simulink model "ex1"  (R2016a)
settings: Solver=ode3  StartTime=0.0  StopTime=inf  FixedStep=0.05  RelTol=1e-3
libraries: dsparch4 x4, simulink x3, vrlib x1, sldrtlib x1
settings Model: ExtModeTrigDuration=100000  Creator=kdle  LastModifiedBy=Khoa
settings DataIOCC: LimitDataPoints=on  SaveFormat=Array
settings DebuggingCC: UnderspecifiedInitializationDetection=Classic  MergeDetectMultiDrivingBlocksExec=none  SolverPrmCheckMsg=warning  StateNameClashWarn=warning
settings HardwareCC: ProdBitPerPointer=32  ProdLargestAtomicFloat=None  ProdIntDivRoundTo=Undefined  ProdEndianess=Unspecified  ProdWordSize=32  ProdHWDeviceType=32-bit Generic
settings ModelReferenceCC: PropagateSignalLabelsOutOfModel=off
settings ConfigComp: CovModelRefEnable=Off

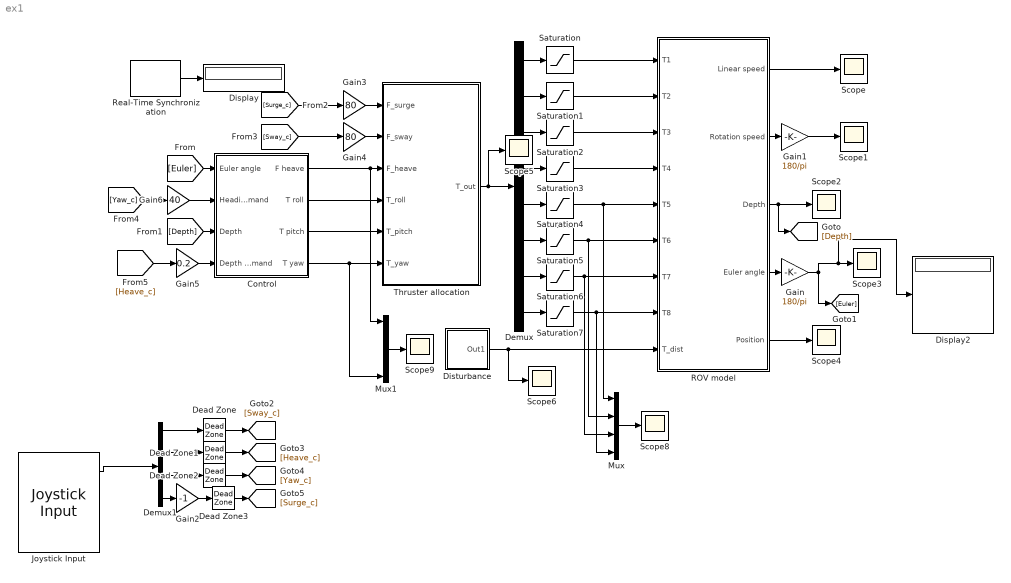
== system ex1 ==
  Control : Subsystem
  Dead Zone{,1..3} (4 alike) : DeadZone  LowerValue=-0.1  UpperValue=0.1  SaturateOnIntegerOverflow=on
  Demux : Demux  Outputs=8
  Demux1 : Demux
  Display : Display
  Display2 : Display
  Disturbance : Subsystem
  Gain : Gain  Gain=180/pi
  Gain1 : Gain  Gain=180/pi
  Gain2 : Gain  Gain=-1
  Gain3 : Gain  Gain=80
  Gain4 : Gain  Gain=80
  Gain5 : Gain  Gain=0.2
  Gain6 : Gain  Gain=40
  Joystick Input : vrlib/Joystick Input  joyid=1  adjustports=on  forcefeed=off
  Mux : Mux
  Mux1 : Mux
  ROV model : Subsystem
  Real-Time Synchronization : sldrtlib/Real-Time Synchronization  SampleTime=0.05  MaxMissedTicks=10000  ShowMissedTicks=on  YieldWhenWaiting=off
  Saturation{,1..3} (4 alike) : Saturate  UpperLimit=50  LowerLimit=-50
  Saturation{4..7} (4 alike) : Saturate  UpperLimit=20  LowerLimit=-20
  Scope{,1..6,8..9} (9 alike) : Scope
  Thruster allocation : MATLAB Function  TreatAsAtomicUnit=on
  wires:
  ROV model/1(Linear speed) -> Scope/1
  ROV model/2(Rotation speed) -> Gain1/1
  ROV model/3(Depth) -> [Depth], Scope2/1
  Disturbance/1(Out1) -> Scope6/1, ROV model/9(T_dist)
  ROV model/4(Euler angle) -> Gain/1
  Thruster allocation/1(T_out) -> Scope5/1, Demux/1
  Demux/7 -> Saturation6/1
  Demux/6 -> Saturation5/1
  Demux/8 -> Saturation7/1
  Demux/5 -> Saturation4/1
  Demux/4 -> Saturation3/1
  Demux/3 -> Saturation2/1
  Demux/2 -> Saturation1/1
  Demux/1 -> Saturation/1
  ROV model/5(Position) -> Scope4/1
  [Euler] -> Control/1(Euler angle)
  [Depth] -> Control/3(Depth)
  [Yaw_c] -> Gain6/1
  [Heave_c] -> Gain5/1
  Gain/1 -> Display2/1, Scope3/1, [Euler]
  Gain1/1 -> Scope1/1
  Saturation/1 -> ROV model/1(T1)
  Saturation1/1 -> ROV model/2(T2)
  Saturation2/1 -> ROV model/3(T3)
  Saturation3/1 -> ROV model/4(T4)
  Saturation4/1 -> Mux/1, ROV model/5(T5)
  Saturation5/1 -> Mux/2, ROV model/6(T6)
  Saturation6/1 -> Mux/3, ROV model/7(T7)
  Saturation7/1 -> Mux/4, ROV model/8(T8)
  Control/1(F heave) -> Mux1/1, Thruster allocation/3(F_heave)
  Control/4(T yaw) -> Mux1/4, Thruster allocation/6(T_yaw)
  Mux/1 -> Scope8/1
  Mux1/1 -> Scope9/1
  Real-Time Synchronization/1 -> Display/1
  Joystick Input/1 -> Demux1/1
  Demux1/1 -> Dead Zone/1
  Demux1/2 -> Dead Zone1/1
  Demux1/3 -> Dead Zone2/1
  Demux1/4 -> Gain2/1
  Gain3/1 -> Thruster allocation/1(F_surge)
  [Surge_c] -> Gain3/1
  [Sway_c] -> Gain4/1
  Gain4/1 -> Thruster allocation/2(F_sway)
  Dead Zone/1 -> [Sway_c]
  Dead Zone1/1 -> [Heave_c]
  Dead Zone2/1 -> [Yaw_c]
  Gain2/1 -> Dead Zone3/1
  Dead Zone3/1 -> [Surge_c]
  Gain5/1 -> Control/4(Depth Command)
  Gain6/1 -> Control/2(Heading Command)
  Control/2(T roll) -> Thruster allocation/4(T_roll)
  Control/3(T pitch) -> Thruster allocation/5(T_pitch)

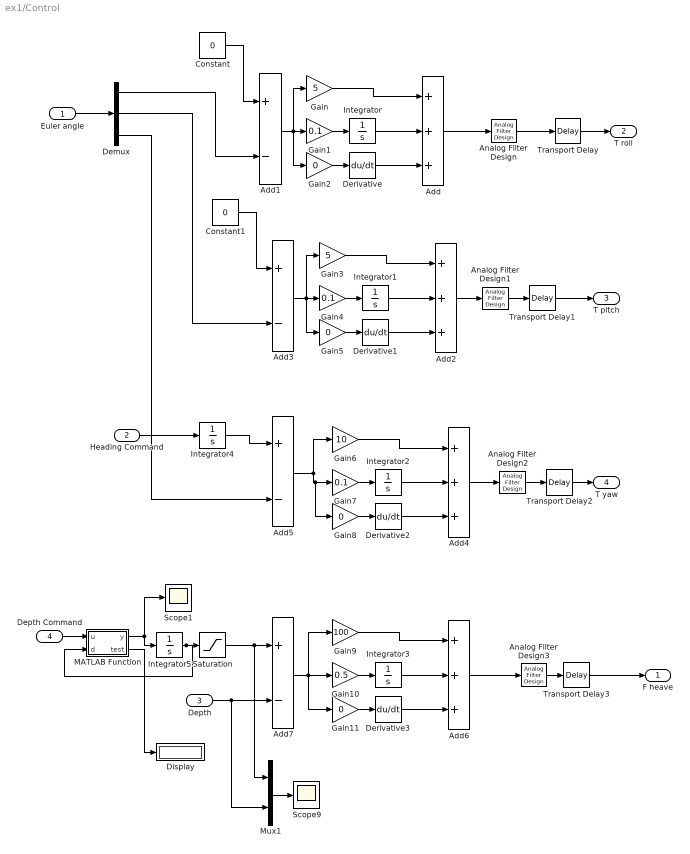
== system ex1/Control ==
  Euler angle : Inport
  Heading Command : Inport  Port=2
  Depth : Inport  Port=3
  Depth Command : Inport  Port=4
  Add{,2,4,6} (4 alike) : Sum  Inputs=+++
  Add{1,3,5,7} (4 alike) : Sum  Inputs=+-
  Analog Filter Design{,1..3} (4 alike) : dsparch4/Analog Filter Design  method=Butterworth  filttype=Lowpass  N=1  Wlo=20  Whi=80  Rp=2  Rs=40
  Constant : Constant  Value=0
  Constant1 : Constant  Value=0
  Demux : Demux  Outputs=3
  Derivative{,1..3} (4 alike) : Derivative
  Display : Display
  Gain : Gain  Gain=5
  Gain1 : Gain  Gain=0.1
  Gain10 : Gain  Gain=0.5
  Gain{2,5,8,11} (4 alike) : Gain  Gain=0
  Gain3 : Gain  Gain=5
  Gain4 : Gain  Gain=0.1
  Gain6 : Gain  Gain=10
  Gain7 : Gain  Gain=0.1
  Gain9 : Gain  Gain=100
  Integrator{,1..4} (5 alike) : Integrator
  Integrator5 : Integrator  InitialCondition=0.01
  MATLAB Function : MATLAB Function  TreatAsAtomicUnit=on
  Mux1 : Mux  Inputs=2
  Saturation : Saturate  UpperLimit=5  LowerLimit=0
  Scope1 : Scope
  Scope9 : Scope
  Transport Delay{,1..3} (4 alike) : TransportDelay  DelayTime=0
  F heave : Outport
  T roll : Outport  Port=2
  T pitch : Outport  Port=3
  T yaw : Outport  Port=4
  wires:
  Euler angle/1 -> Demux/1
  Gain1/1 -> Integrator/1
  Gain2/1 -> Derivative/1
  Gain/1 -> Add/1
  Integrator/1 -> Add/2
  Derivative/1 -> Add/3
  Add1/1 -> Gain2/1, Gain/1, Gain1/1
  Demux/1 -> Add1/2
  Constant/1 -> Add1/1
  Add/1 -> Analog Filter Design/1
  Gain4/1 -> Integrator1/1
  Gain5/1 -> Derivative1/1
  Gain3/1 -> Add2/1
  Integrator1/1 -> Add2/2
  Derivative1/1 -> Add2/3
  Add3/1 -> Gain4/1, Gain3/1, Gain5/1
  Demux/2 -> Add3/2
  Constant1/1 -> Add3/1
  Add2/1 -> Analog Filter Design1/1
  Gain7/1 -> Integrator2/1
  Gain8/1 -> Derivative2/1
  Gain6/1 -> Add4/1
  Integrator2/1 -> Add4/2
  Derivative2/1 -> Add4/3
  Gain10/1 -> Integrator3/1
  Gain11/1 -> Derivative3/1
  Gain9/1 -> Add6/1
  Integrator3/1 -> Add6/2
  Derivative3/1 -> Add6/3
  Add6/1 -> Analog Filter Design3/1
  Analog Filter Design/1 -> Transport Delay/1
  Analog Filter Design1/1 -> Transport Delay1/1
  Analog Filter Design2/1 -> Transport Delay2/1
  Analog Filter Design3/1 -> Transport Delay3/1
  Add4/1 -> Analog Filter Design2/1
  Transport Delay/1 -> T roll/1
  Transport Delay1/1 -> T pitch/1
  Transport Delay2/1 -> T yaw/1
  Transport Delay3/1 -> F heave/1
  Add5/1 -> Gain6/1, Gain8/1, Gain7/1
  Add7/1 -> Gain11/1, Gain9/1, Gain10/1
  Demux/3 -> Add5/2
  Heading Command/1 -> Integrator4/1
  Integrator4/1 -> Add5/1
  Depth/1 -> Mux1/2, Add7/2
  MATLAB Function/1(y) -> Integrator5/1, Scope1/1
  Depth Command/1 -> MATLAB Function/1(u)
  Integrator5/1 -> MATLAB Function/2(d), Saturation/1
  Mux1/1 -> Scope9/1
  Saturation/1 -> Mux1/1, Add7/1
  MATLAB Function/2(test) -> Display/1

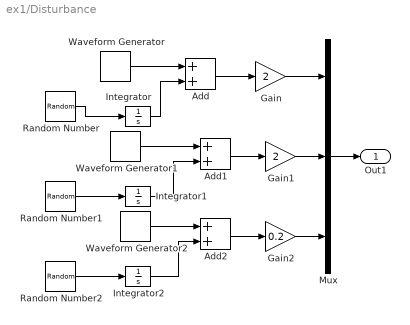
== system ex1/Disturbance ==
  Add : Sum
  Add1 : Sum
  Add2 : Sum
  Gain : Gain  Gain=2
  Gain1 : Gain  Gain=2
  Gain2 : Gain  Gain=0.2
  Integrator : Integrator
  Integrator1 : Integrator
  Integrator2 : Integrator
  Mux : Mux  Inputs=3
  Random Number : RandomNumber  Variance=4
  Random Number1 : RandomNumber  Variance=3.5  Seed=19
  Random Number2 : RandomNumber  Variance=2.7  Seed=12
  Waveform Generator : simulink/Sources/Waveform Generator  OutMin=[]  OutMax=[]  OutDataTypeStr=double  SelectedSignal=1  Signals=sin(9,0.8,1)+sin(3,1,90)+sin(0.5,2.3,150)#  BlockNames=MultiportSwitch_466ab8b035bb466#MultiportSwitch_63944deda71346d  SampleTime=-1
  Waveform Generator1 : simulink/Sources/Waveform Generator  OutMin=[]  OutMax=[]  OutDataTypeStr=double  SelectedSignal=1  Signals=sin(10,0.9,-80)+sin(3.5,1.2,90)+sin(0.5,2,180)##  BlockNames=MultiportSwitch_830e07a5a85d43f#MultiportSwitch_1fa4dfc1fb8347c#MultiportSwitch_a18988079fe14e6  SampleTime=-1
  Waveform Generator2 : simulink/Sources/Waveform Generator  OutMin=[]  OutMax=[]  OutDataTypeStr=double  SelectedSignal=1  Signals=sin(7,1.1,-80)+sin(3.4,1.6,85)+sin(0.5,2,180)##  BlockNames=MultiportSwitch_b1ec6a342e4a44b#MultiportSwitch_f195588b21b946e#MultiportSwitch_f4c491ab188140c  SampleTime=-1
  Out1 : Outport
  wires:
  Mux/1 -> Out1/1
  Waveform Generator/1 -> Add/1
  Add/1 -> Gain/1
  Add1/1 -> Gain1/1
  Waveform Generator1/1 -> Add1/1
  Add2/1 -> Gain2/1
  Waveform Generator2/1 -> Add2/1
  Random Number/1 -> Integrator/1
  Random Number1/1 -> Integrator1/1
  Random Number2/1 -> Integrator2/1
  Integrator/1 -> Add/2
  Integrator1/1 -> Add1/2
  Integrator2/1 -> Add2/2
  Gain/1 -> Mux/1
  Gain1/1 -> Mux/2
  Gain2/1 -> Mux/3

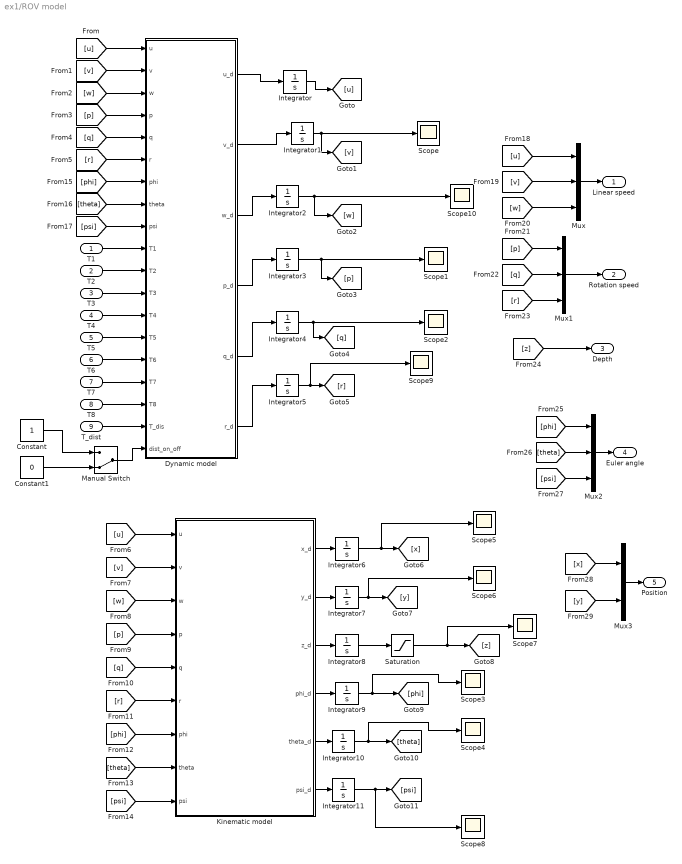
== system ex1/ROV model ==
  T1 : Inport
  T2 : Inport  Port=2
  T3 : Inport  Port=3
  T4 : Inport  Port=4
  T5 : Inport  Port=5
  T6 : Inport  Port=6
  T7 : Inport  Port=7
  T8 : Inport  Port=8
  T_dist : Inport  Port=9
  Constant : Constant
  Constant1 : Constant  Value=0
  Dynamic model : MATLAB Function  TreatAsAtomicUnit=on
  Integrator{,1..11} (12 alike) : Integrator
  Kinematic model : MATLAB Function  TreatAsAtomicUnit=on
  Manual Switch : ManualSwitch  CurrentSetting=0
  Mux : Mux  Inputs=3
  Mux1 : Mux  Inputs=3
  Mux2 : Mux  Inputs=3
  Mux3 : Mux  Inputs=2
  Saturation : Saturate  UpperLimit=5  LowerLimit=0
  Scope{,1..10} (11 alike) : Scope
  Linear speed : Outport
  Rotation speed : Outport  Port=2
  Depth : Outport  Port=3
  Euler angle : Outport  Port=4
  Position : Outport  Port=5
  wires:
  T1/1 -> Dynamic model/10(T1)
  T2/1 -> Dynamic model/11(T2)
  T3/1 -> Dynamic model/12(T3)
  Dynamic model/1(u_d) -> Integrator/1
  Dynamic model/2(v_d) -> Integrator1/1
  Dynamic model/3(w_d) -> Integrator2/1
  Dynamic model/4(p_d) -> Integrator3/1
  Dynamic model/5(q_d) -> Integrator4/1
  Dynamic model/6(r_d) -> Integrator5/1
  Integrator/1 -> [u]
  Integrator1/1 -> [v], Scope/1
  Integrator2/1 -> [w], Scope10/1
  Integrator3/1 -> [p], Scope1/1
  Integrator4/1 -> [q], Scope2/1
  Integrator5/1 -> Scope9/1, [r]
  [u] -> Dynamic model/1(u)
  [v] -> Dynamic model/2(v)
  [w] -> Dynamic model/3(w)
  [p] -> Dynamic model/4(p)
  [r] -> Dynamic model/6(r)
  [q] -> Dynamic model/5(q)
  [u] -> Kinematic model/1(u)
  [r] -> Kinematic model/6(r)
  [q] -> Kinematic model/5(q)
  [p] -> Kinematic model/4(p)
  [w] -> Kinematic model/3(w)
  [v] -> Kinematic model/2(v)
  Kinematic model/1(x_d) -> Integrator6/1
  Kinematic model/2(y_d) -> Integrator7/1
  Kinematic model/3(z_d) -> Integrator8/1
  Kinematic model/4(phi_d) -> Integrator9/1
  Kinematic model/5(theta_d) -> Integrator10/1
  Kinematic model/6(psi_d) -> Integrator11/1
  Integrator6/1 -> Scope5/1, [x]
  Integrator7/1 -> Scope6/1, [y]
  Integrator8/1 -> Saturation/1
  Integrator9/1 -> Scope3/1, [phi]
  Integrator10/1 -> Scope4/1, [theta]
  Integrator11/1 -> Scope8/1, [psi]
  [phi] -> Kinematic model/7(phi)
  [theta] -> Kinematic model/8(theta)
  [psi] -> Kinematic model/9(psi)
  [phi] -> Dynamic model/7(phi)
  [theta] -> Dynamic model/8(theta)
  T4/1 -> Dynamic model/13(T4)
  T5/1 -> Dynamic model/14(T5)
  T6/1 -> Dynamic model/15(T6)
  T7/1 -> Dynamic model/16(T7)
  T8/1 -> Dynamic model/17(T8)
  [psi] -> Dynamic model/9(psi)
  T_dist/1 -> Dynamic model/18(T_dis)
  [u] -> Mux/1
  [v] -> Mux/2
  [w] -> Mux/3
  Mux/1 -> Linear speed/1
  [p] -> Mux1/1
  [q] -> Mux1/2
  [r] -> Mux1/3
  Mux1/1 -> Rotation speed/1
  [z] -> Depth/1
  Mux2/1 -> Euler angle/1
  [phi] -> Mux2/1
  [theta] -> Mux2/2
  [psi] -> Mux2/3
  Mux3/1 -> Position/1
  [x] -> Mux3/1
  [y] -> Mux3/2
  Saturation/1 -> Scope7/1, [z]
  Manual Switch/1 -> Dynamic model/19(dist_on_off)
  Constant/1 -> Manual Switch/1
  Constant1/1 -> Manual Switch/2

== matlab function ex1/ROV model/Kinematic model ==
  data: u input; v input; w input; p input; q input; r input; x_d output; y_d output; z_d output; phi_d output; theta_d output; psi_d output; phi input; theta input; psi input
function [x_d,y_d,z_d,phi_d,theta_d,psi_d] = fcn(u,v,w,p,q,r,phi,theta,psi)
% Jacobian matrix
J=zeros(6,6);
% rotational matrix
J(1,1)=cos(psi)*cos(theta);
J(1,2)=-sin(psi)*cos(phi)+cos(psi)*sin(theta)*sin(phi);
J(1,3)=sin(psi)*sin(phi)+cos(psi)*cos(phi)*sin(theta);
J(2,1)=sin(psi)*cos(theta);
J(2,2)=cos(psi)*cos(phi)+sin(phi)*sin(theta)*sin(psi);
J(2,3)=-cos(psi)*sin(phi)+sin(theta)*sin(psi)*cos(phi);
J(3,1)=-sin(theta);
J(3,2)=cos(theta)*sin(phi);
J(3,3)=cos(theta)*cos(phi);

% transformation matrix
J(4,4)=1;
J(4,5)=sin(phi)*tan(theta);
J(4,6)=cos(phi)*tan(theta);
J(5,5)=cos(phi);
J(5,6)=-sin(phi);
J(6,5)=sin(phi)/cos(theta);
J(6,6)=cos(phi)/cos(theta);

% Local velocity vectors
L_V=[u v w p q r]';

% Output matrix
G_V=zeros(6,1);
G_V=J*L_V;

% Output results
x_d=G_V(1,1);
y_d=G_V(2,1);
z_d=G_V(3,1);
phi_d=G_V(4,1);
theta_d=G_V(5,1);
psi_d=G_V(6,1);

== matlab function ex1/ROV model/Dynamic model ==
  data: u input; v input; w input; p input; q input; r input; phi input; theta input; psi input; T1 input; u_d output; T2 input; T3 input; v_d output; w_d output; p_d output; q_d output; r_d output; T4 input; T5 input; T6 input; T7 input; T8 input; T_dis input; dist_on_off input
function [u_d,v_d,w_d,p_d,q_d,r_d] = fcn(u,v,w,p,q,r,phi,theta, psi,T1,T2,T3,T4,T5,T6,T7,T8,T_dis,dist_on_off)
% mass of the system
m=50;
% Moment of inertia
Ix=6.3;Iy=7.8;Iz=3.24;
% assumet that the other elements of moment inertia are zero
Ixy=0.21;Ixz=0.13;Iyz=0.11;
% added mass parameter
X_ud=16.66;Y_vd=20.43;Z_wd=30.78;
K_pd=2.35;M_qd=3.75;N_rd=4.84;
% Linear damping coefficient
X_u=4.89;Y_v=4.96;Z_w=9.25;K_p=8.71;M_q=9.91;N_r=10.81;
% Quadratic damping
X_au=250.3;Y_av=250.4;Z_aw=350.37;K_ap=260.2;M_aq=290.1;N_ar=250.4;
% distance
d=0.25;

% Position of buoyancy center
xB=-0.02; yB=0.00;
zB=-0.05;

% Position of gravity center
xg=0.00;yg=-0.00;zg=0.00;

%Buyancy force with assumption B=W
B=500;



% Inertia matrix
M=zeros(6,6);
% Coriolis matrix
C=zeros(6,6);
% Damping matix
D=zeros(6,6);

%Rigid body inertia matrix
M_rb=zeros(6,6);
% Row 1
M_rb(1,1)=m;
M_rb(1,5)=m*zg;
M_rb(1,6)=-m*yg;
% Row 2
M_rb(2,2)=m;
M_rb(2,4)=-m*zg;
M_rb(2,6)=m*xg;
% Row 3
M_rb(3,3)=m;
M_rb(3,4)=m*yg;
M_rb(3,5)=-m*xg;
% Row 4
M_rb(4,2)=-m*zg;
M_rb(4,3)=m*yg;
M_rb(4,4)=Ix;
M_rb(4,5)=-Ixy;
M_rb(4,6)=-Ixz;
% Row 5
M_rb(5,1)=m*zg;
M_rb(5,3)=-m*xg;
M_rb(5,4)=-Ixy;
M_rb(5,5)=Iy;
M_rb(5,6)=-Iyz;
% Row 6
M_rb(6,1)=-m*yg;
M_rb(6,2)=m*xg;
M_rb(6,4)=-Ixz;
M_rb(6,5)=-Iyz;
M_rb(6,6)=Iz;

% Added mass matrix
M_a=zeros(6,6);
M_a(1,1)=X_ud;M_a(2,2)=Y_vd;M_a(3,3)=Z_wd;M_a(4,4)=K_pd;M_a(5,5)=M_qd;M_a(6,6)=N_rd;
% Inertia matrix
M=M_rb+M_a;

%Coriolis of rigid body
C_rb=zeros(6,6);
% row 1
C_rb(1,2)=-m*r;
C_rb(1,3)=m*q;
% row 2
C_rb(2,1)=m*r;
C_rb(2,3)=-m*p;
% row 3
C_rb(3,1)=-m*q;
C_rb(3,2)=m*p;
% row 4
C_rb(4,5)=Iz*r;
C_rb(4,6)=-Iy*q;
% row 5
C_rb(5,4)=-Ix*r;
C_rb(5,6)=Iz*p;
% row 6
C_rb(6,4)=Iy*q;
C_rb(6,5)=-Ix*p;

% Coriolis of added mass
C_a=zeros(6,6);
% Rox 1
C_a(1,5)=-Z_wd*w;
C_a(1,6)=Y_vd*v;
% Rox 2
C_a(2,4)=Z_wd*w;
C_a(2,6)=-X_ud*u;
% Rox 3
C_a(3,4)=-Y_vd*v;
C_a(3,5)=X_ud*u;
% Rox 4
C_a(4,2)=-Z_wd*w;
C_a(4,3)=Y_vd*v;
C_a(4,5)=-N_rd*r;
C_a(4,6)=M_qd*q;
% Rox 5
C_a(5,1)=Z_wd*w;
C_a(5,3)=-X_ud*u;
C_a(5,4)=N_rd*r;
C_a(5,6)=-K_pd*p;
% Rox 6
C_a(6,1)=-Y_vd*v;
C_a(6,2)=X_ud*u;
C_a(6,4)=-M_qd*q;
C_a(6,5)=K_pd*p;

% Coriolis matrix
C=C_rb+C_a;

% Damping matrix
D(1,1)=X_u+X_au*abs(u);
D(2,2)=Y_v+Y_av*abs(v);
D(3,3)=Z_w+Z_aw*abs(w);
D(4,4)=K_p+K_ap*abs(p);
D(5,5)=M_q+M_aq*abs(q);
D(6,6)=N_r+N_ar*abs(r);

% Restoring force
g=zeros(6,1);
g(4,1)=-zB*B*cos(theta)*sin(phi) + yB*B*cos(theta)*cos(phi);
% g(4,1)=0;
g(5,1)=-zB*B*sin(theta)-xB*B*cos(theta)*cos(phi);
g(6,1)=xB*B*cos(theta)*sin(phi) + yB*B*sin(theta);


% disturbance
J=zeros(3,3);
J(1,1)=cos(psi)*cos(theta);
J(1,2)=-sin(psi)*cos(phi)+cos(psi)*sin(theta)*sin(phi);
J(1,3)=sin(psi)*sin(phi)+cos(psi)*cos(phi)*sin(theta);
J(2,1)=sin(psi)*cos(theta);
J(2,2)=cos(psi)*cos(phi)+sin(phi)*sin(theta)*sin(psi);
J(2,3)=-cos(psi)*sin(phi)+sin(theta)*sin(psi)*cos(phi);
J(3,1)=-sin(theta);
J(3,2)=cos(theta)*sin(phi);
J(3,3)=cos(theta)*cos(phi);

current_l=zeros(1,3);
current_g=[4 -20 1]';
current_l=(J^-1)*current_g;
if (dist_on_off==1)
   k_dist=1; % disturbance gain
else
    k_dist=0;
end
% Input force
T=zeros(6,1);
% Surge force
T(1,1)=(T1+T2+T3+T4)/sqrt(2) + (current_l(1)+rand*3)*k_dist;

% Sway force
T(2,1)=(T1-T2+T3-T4)/sqrt(2)+ (current_l(2)+rand*3)*k_dist;

% Heave force;
T(3,1)=(T5+T6+T7+T8) + (current_l(3)+rand*5)*k_dist;

% Dimension of ROV length a, width b
a=0.85;
b=0.58;
% Roll moment
% T(4,1)=(T5-T6-T7+T8)*b/2 + T_dis(1)*k_dist ;
T(4,1)=T5*(b/2+yg)-T6*(b/2-yg)-T7*(b/2-yg)+T8*(b/2+yg) + zg*(T1-T2-T3+T4)*sqrt(a^2+b^2)/2 +T_dis(1)*k_dist ;
% Pitch moment
% T(5,1)=(T5+T6-T7-T8)*a/2 + T_dis(2)*k_dist;
T(5,1)=T5*(a/2-xg)+T6*(a/2-xg)-T7*(a/2+xg)-T8*(a/2+xg) +zg*(T1-T2-T3+T4)*sqrt(a^2+b^2)/2+ T_dis(2)*k_dist;

% Yaw momend
T(6,1)=(T1-T2-T3+T4)*sqrt(a^2+b^2)/2+ T_dis(3)*k_dist ;


%  T=zeros(6,1);
% T(1,1)=T1+T2; % Surge force
% T(3,1)=T3;    % heave force
% T(5,1)=0.1*(T1+T2)-0*T3; % coupling force
% T(6,1)=d*(T1-T2); % yaw moment

% velocity vector
V=[u v w p q r]';

% Right handside matrix
 R_M=T-C*V-D*V-g;
%   R_M=T-D*V-g;

% Accelerometer
V_d=zeros(6,1);
V_d=(M^-1)*R_M;

% output value

u_d=V_d(1,1);
v_d=V_d(2,1);
w_d=V_d(3,1);
p_d=V_d(4,1);
q_d=V_d(5,1);
r_d=V_d(6,1);

== matlab function ex1/Thruster allocation ==
  data: F_surge input; T_out output; F_sway input; F_heave input; T_roll input; T_pitch input; T_yaw input
function T_out = fcn(F_surge,F_sway,F_heave,T_roll,T_pitch,T_yaw)
T_out=zeros(1,8);
% Dimension of ROV
a=0.8;
b=0.6;
D=sqrt(a^2+b^2);
OUT=zeros(1,8);
% Allocation matix

a1=1/sqrt(2);

M=[a1  a1 a1  a1 0   0    0    0;
   a1 -a1 a1 -a1 0   0    0    0;
    0  0  0   0  1   1    1    1;
    0  0  0   0  b/2 -b/2 -b/2 b/2;
    0  0  0   0  a/2 a/2  -a/2 -a/2;
    D  -D  -D D  0   0     0    0];

IN=[F_surge F_sway F_heave T_roll T_pitch T_yaw]';
In_M=M'*((M*M')^-1);
OUT=In_M*IN;
for i=1:length(OUT)
    T_out(i)=OUT(i);
end

== matlab function ex1/Control/MATLAB Function ==
  data: u input; y output; d input; test output
function [y,test] = fcn(u,d)
if ((d>=5) && (u>0))
    y=0;
    test=0;
elseif ((d<=0) && (u<0))
    y=0;
    test=0;
else
    y=u;
    test=1;
end
